simulink model "motor_dtf_step_double"  (R2021b)
settings: Solver=FixedStepDiscrete  StartTime=0.0  StopTime=120  RelTol=1e-3
undefined symbols (not defined in the file): DiscIntNeverNeededParam
Description:
  | Symmetric FIR Filter
  | This example shows how to use HDL Coder(TM) to check, generate,
  | and verify HDL for a fixed-point symmetric FIR filter.
settings Model: DataTypeOverride=Off  Creator=The MathWorks, Inc.  LastModifiedBy=Marco Milanesi
settings SolverCC: AlgebraicLoopSolver=TrustRegion  AutoInsertRateTranBlk=on
settings DataIOCC: LimitDataPoints=on  SaveFormat=Array  SaveOutput=off  SignalLogging=off  SaveTime=off  ReturnWorkspaceOutputs=off  SignalLoggingName=logsOut
settings OptimizationCC: BlockReduction=off  BooleanDataType=off  ConditionallyExecuteInputs=off  DefaultParameterBehavior=Inlined  InheritOutputTypeSmallerThanSingle=on  InlineInvariantSignals=on  ExpressionDepthLimit=2147483647  InitFltsAndDblsToZero=on  LifeSpan=inf  BufferReusableBoundary=off
settings DebuggingCC: AlgebraicLoopMsg=error  SaveWithParameterizedLinksMsg=none  UnderspecifiedInitializationDetection=Classic  MergeDetectMultiDrivingBlocksExec=none  CheckExecutionContextPreStartOutputMsg=on  SignalResolutionControl=TryResolveAllWithWarning  MultiTaskDSMMsg=warning  MultiTaskCondExecSysMsg=none  SingleTaskRateTransMsg=error  IntegerOverflowMsg=none  ParameterPrecisionLossMsg=none  FcnCallInpInsideContextMsg=warning  BusObjectLabelMismatch=none  StateNameClashWarn=warning  SFUnexpectedBacktrackingDiag=warning  SFNoUnconditionalDefaultTransitionDiag=warning  SFExecutionAtInitializationDiag=none  SFMachineParentedDataDiag=warning  IntegerSaturationMsg=none  ArithmeticOperatorsInVariantConditions=warning
settings HardwareCC: ProdBitPerPointer=32  ProdBitPerSizeT=32  ProdBitPerPtrDiffT=32  ProdLargestAtomicFloat=None  ProdIntDivRoundTo=Undefined  ProdEndianess=Unspecified  ProdWordSize=32  ProdHWDeviceType=ASIC/FPGA  TargetUnknown=on  ProdEqTarget=off
settings ModelReferenceCC: PropagateSignalLabelsOutOfModel=off
settings SFSimCC: SimUseLocalCustomCode=off  CustomCodeUndefinedFunction=UseInterfaceOnly
settings RTWCC: RTWUseLocalCustomCode=off
settings CodeAppCC: StateflowObjectComments=on
settings GRTTargetCC: TargetFcnLib=ansi_tfl_tmw.mat  TargetLangStandard=C89/C90 (ANSI)  CombineOutputUpdateFcns=off  GRTInterface=on
settings ConfigComp: CovMetricSettings=dw  CovSaveCumulativeToWorkspaceVar=on  CovSaveSingleToWorkspaceVar=on  CovExternalEMLEnable=off

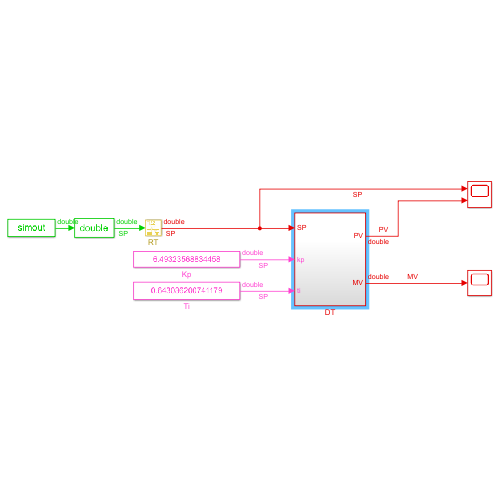
[thumbnail: Simulink's stored preview of the top-level diagram]
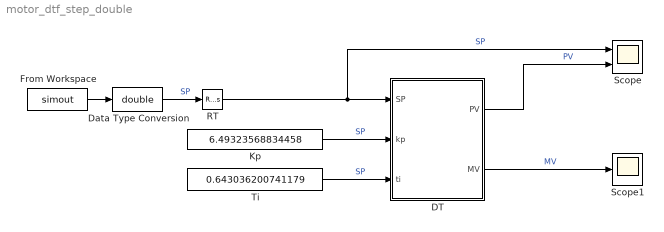
== system motor_dtf_step_double ==
  DT : Subsystem
  Data Type Conversion : DataTypeConversion  OutDataTypeStr=double
  From Workspace : FromWorkspace  VariableName=simout  SampleTime=1  OutputAfterFinalValue=Setting to zero
  Kp : Constant  Value=6.49323568834458
  RT : RateTransition  OutPortSampleTime=0.001
  Scope : Scope  NumInputPorts=2
  Scope1 : Scope
  Ti : Constant  Value=0.643036200741179
  wires:
  DT/1(PV) -> Scope/2  "PV"
  From Workspace/1 -> Data Type Conversion/1
  DT/2(MV) -> Scope1/1  "MV"
  Kp/1 -> DT/2(kp)  "SP"
  Ti/1 -> DT/3(ti)  "SP"
  RT/1 -> Scope/1, DT/1(SP)  "SP"
  Data Type Conversion/1 -> RT/1  "SP"

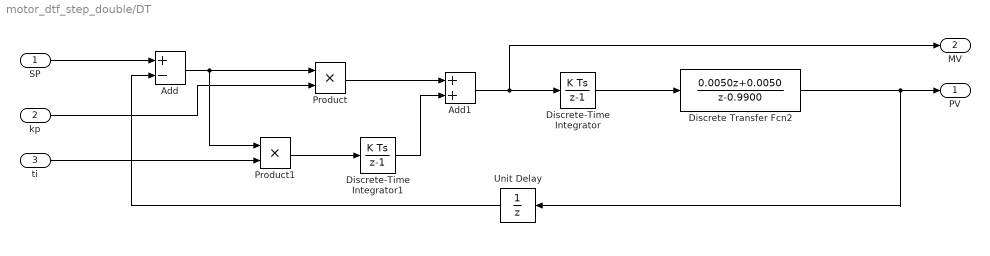
== system motor_dtf_step_double/DT ==
  SP : Inport
  kp : Inport  Port=2
  ti : Inport  Port=3
  Add : Sum  Inputs=+-  AccumDataTypeStr=double  OutDataTypeStr=double
  Add1 : Sum  AccumDataTypeStr=double  OutDataTypeStr=double
  Discrete Transfer Fcn2 : DiscreteTransferFcn  Numerator=[0.0050 0.0050]  Denominator=[1 -0.9900]  OutDataTypeStr=Inherit: Same as input
  Discrete-Time Integrator : DiscreteIntegrator  SampleTime=-1  OutDataTypeStr=double  ICPrevOutput=DiscIntNeverNeededParam  ICPrevScaledInput=DiscIntNeverNeededParam
  Discrete-Time Integrator1 : DiscreteIntegrator  SampleTime=-1  OutDataTypeStr=double  ICPrevOutput=DiscIntNeverNeededParam  ICPrevScaledInput=DiscIntNeverNeededParam
  Product : Product  OutDataTypeStr=double
  Product1 : Product  OutDataTypeStr=double
  Unit Delay : UnitDelay  SampleTime=0.001  HasFrameUpgradeWarning=on
  PV : Outport  VectorParamsAs1DForOutWhenUnconnected=off
  MV : Outport  Port=2  VectorParamsAs1DForOutWhenUnconnected=off
  wires:
  SP/1 -> Add/1
  Discrete Transfer Fcn2/1 -> Unit Delay/1, PV/1
  Add/1 -> Product/1, Product1/1
  kp/1 -> Product/2
  Product/1 -> Add1/1
  ti/1 -> Product1/2
  Product1/1 -> Discrete-Time Integrator1/1
  Discrete-Time Integrator1/1 -> Add1/2
  Add1/1 -> MV/1, Discrete-Time Integrator/1
  Discrete-Time Integrator/1 -> Discrete Transfer Fcn2/1
  Unit Delay/1 -> Add/2
